simulink model "all_phase_inv"  (Simulink 4.00)
settings: Solver=ode45  StartTime=0.0  StopTime=0.5  RelTol=1e-3
settings Model: LastModifiedBy=dev  BlockReductionOpt=off

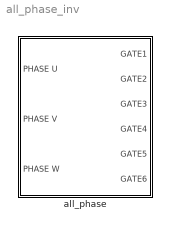
== system all_phase_inv ==
  all_phase : Subsystem  Orientation=left  mask{BV=1}
      mask prompts: BV "Battery voltage for excitation"
      mask help: This is an inverter. Double click the block to enter the battery voltage
      settings: RTWFcnNameOpts=Auto  RTWFileNameOpts=Auto

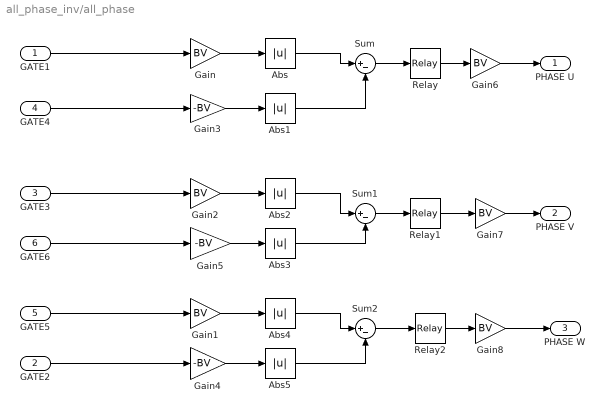
== system all_phase_inv/all_phase ==
  GATE1 : Inport  Port=1
  GATE2 : Inport  Port=2
  GATE3 : Inport  Port=3
  GATE4 : Inport  Port=4
  GATE5 : Inport  Port=5
  GATE6 : Inport  Port=6
  Abs{,1..5} (6 alike) : Abs  SaturateOnIntegerOverflow=on
  Gain{,1..2,6..8} (6 alike) : Gain  Gain=BV  Multiplication=Element-wise(K.*u)  SaturateOnIntegerOverflow=on
  Gain3 : Gain  Gain=-BV  Multiplication=Element-wise(K.*u)  SaturateOnIntegerOverflow=on
  Gain4 : Gain  Gain=-BV  Multiplication=Element-wise(K.*u)  SaturateOnIntegerOverflow=on
  Gain5 : Gain  Gain=-BV  Multiplication=Element-wise(K.*u)  SaturateOnIntegerOverflow=on
  Relay : Relay  OnSwitchValue=0  OffSwitchValue=0  OnOutputValue=1  OffOutputValue=0
  Relay1 : Relay  OnSwitchValue=0  OffSwitchValue=0  OnOutputValue=1  OffOutputValue=0
  Relay2 : Relay  OnSwitchValue=0  OffSwitchValue=0  OnOutputValue=1  OffOutputValue=0
  Sum : Sum  Inputs=|+-  SaturateOnIntegerOverflow=on
  Sum1 : Sum  Inputs=|+-  SaturateOnIntegerOverflow=on
  Sum2 : Sum  Inputs=|+-  SaturateOnIntegerOverflow=on
  PHASE U : Outport  Port=1
  PHASE V : Outport  Port=2
  PHASE W : Outport  Port=3
  wires:
  GATE1/1 -> Gain/1
  GATE5/1 -> Gain1/1
  GATE3/1 -> Gain2/1
  GATE4/1 -> Gain3/1
  GATE2/1 -> Gain4/1
  GATE6/1 -> Gain5/1
  Gain/1 -> Abs/1
  Gain3/1 -> Abs1/1
  Gain2/1 -> Abs2/1
  Gain5/1 -> Abs3/1
  Gain1/1 -> Abs4/1
  Gain4/1 -> Abs5/1
  Abs/1 -> Sum/1
  Abs1/1 -> Sum/2
  Abs2/1 -> Sum1/1
  Abs3/1 -> Sum1/2
  Abs4/1 -> Sum2/1
  Abs5/1 -> Sum2/2
  Sum/1 -> Relay/1
  Relay/1 -> Gain6/1
  Sum1/1 -> Relay1/1
  Relay1/1 -> Gain7/1
  Sum2/1 -> Relay2/1
  Relay2/1 -> Gain8/1
  Gain8/1 -> PHASE W/1
  Gain7/1 -> PHASE V/1
  Gain6/1 -> PHASE U/1
